simulink model "buck_N"  (R2023a)
settings: Solver=ode4  StartTime=0.0  StopTime=Tsin  FixedStep=Ts  RelTol=1e-3
values from neighbouring files (symbols this model uses):
  C1 = 100e-6*(1.0)    (= 0.0001)    [ripp_buck2.m]
  kd = x3    [ripp_buck2.m]
  ki = x2    [ripp_buck2.m]
  kp = x1    [ripp_buck2.m]
  L1 = 1e-3*(1.0)    (= 0.001)    [ripp_buck2.m]
  R1 = 6    [ripp_buck2.m]
  Ref = 3    [ripp_buck2.m]
  Ts = H.SettlingTime    [HHbuck.m]    (also in ripp_buck2.m)
  Tsin = 0.01    [ripp_buck2.m]
  Vg = 36    [ripp_buck2.m]
libraries: simulink x3, spsSeriesRLCBranchLib x3, spsControlledCurrentSourceLib x1, spsCurrentMeasurementLib x1, spsDCVoltageSourceLib x1, spsDiodeLib x1, spsMosfetLib x1, spsPWMGeneratorDCDCLib x1, spsVoltageMeasurementLib x1, spspowerguiLib x1
settings Model: SimulationMode=accelerator  Creator=danie  LastModifiedBy=Daniel
settings DataIOCC: ReturnWorkspaceOutputs=off
settings ModelReferenceCC: EnableRefExpFcnMdlSchedulingChecks=on

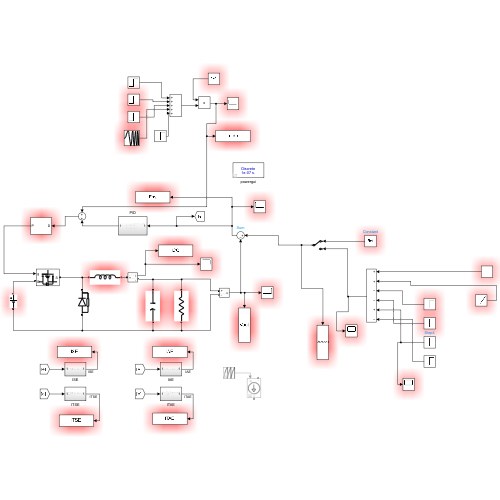
[thumbnail: Simulink's stored preview of the top-level diagram]
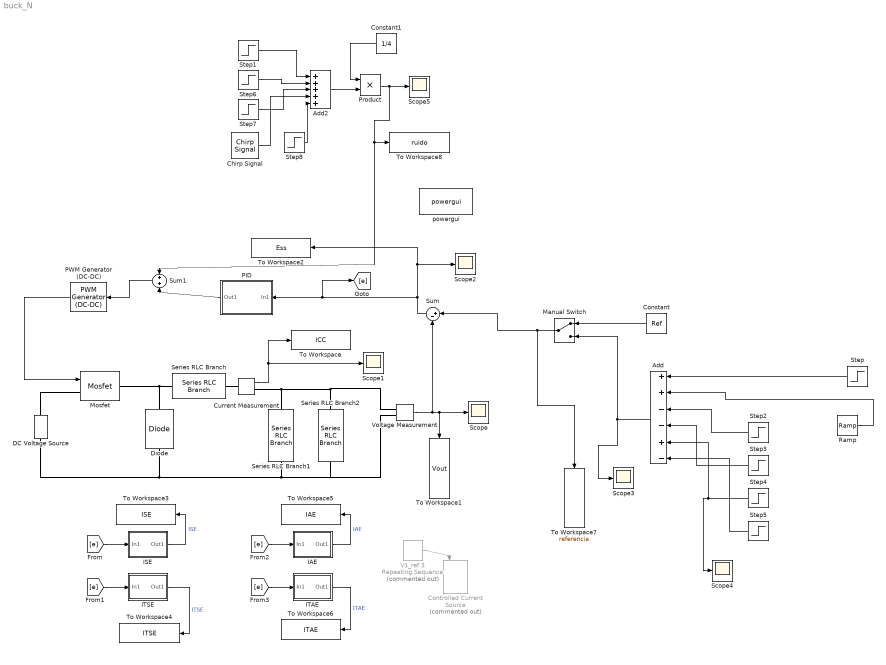
== system buck_N ==
  Add : Sum  Inputs=++--+-
  Add2 : Sum  Inputs=+++++
  Chirp Signal : simulink/Sources/Chirp Signal  f1=1e2  T=Tsin  f2=5e3
  Constant : Constant  Value=Ref  SampleTime=Ts
  Constant1 : Constant  Value=1/4  SampleTime=Ts
  Controlled Current Source : spsControlledCurrentSourceLib/Controlled Current Source  Commented=on  Initialize=off  Source_Type=AC  Amplitude=0  Phase=0  Frequency=0  Measurements=None
  Current Measurement : spsCurrentMeasurementLib/Current Measurement  PhasorSimulation=off  OutputType=Complex  PSBequivalent=0
  DC Voltage Source : spsDCVoltageSourceLib/DC Voltage Source  Amplitude=Vg  Measurements=None
  Diode : spsDiodeLib/Diode  Ron=0.001  Lon=0  Vf=0.8  IC=0  UseSnubber=0  Rs=500  Cs=250e-9  Measurements=off
  IAE : Subsystem
  ISE : Subsystem
  ITAE : Subsystem
  ITSE : Subsystem
  Manual Switch : ManualSwitch
  Mosfet : spsMosfetLib/Mosfet  Ron=0.1  Lon=0  Rd=0.01  Vfd=0  IC=0  Rs=1e5  Cs=inf  Measurements=off
  PID : Subsystem
  PWM Generator (DC-DC) : spsPWMGeneratorDCDCLib/PWM Generator (DC-DC)  Fsw=F  Ts=Ts
  Product : Product
  Ramp : simulink/Sources/Ramp  slope=100  start=Tsin/2  InitialOutput=0
  Scope{,1..5} (6 alike) : Scope
  Series RLC Branch : spsSeriesRLCBranchLib/Series RLC Branch  LConnTagsString=__new0  RConnTagsString=__new0  BranchType=L  Resistance=1  Inductance=L1  SetiL0=off  InitialCurrent=0  Capacitance=1e-6  Setx0=off  InitialVoltage=0  Measurements=None
  Series RLC Branch1 : spsSeriesRLCBranchLib/Series RLC Branch  LConnTagsString=__new0  RConnTagsString=__new0  BranchType=C  Resistance=1  Inductance=1e-3  SetiL0=off  InitialCurrent=0  Capacitance=C1  Setx0=off  InitialVoltage=0  Measurements=None
  Series RLC Branch2 : spsSeriesRLCBranchLib/Series RLC Branch  LConnTagsString=__new0  RConnTagsString=__new0  BranchType=R  Resistance=R1  Inductance=1e-3  SetiL0=off  InitialCurrent=0  Capacitance=1e-6  Setx0=off  InitialVoltage=0  Measurements=None
  Step : Step  Time=Tsin/5  After=3  SampleTime=0
  Step1 : Step  Time=0  After=0.5  SampleTime=0
  Step2 : Step  Time=Tsin/3  After=2  SampleTime=0
  Step3 : Step  Time=Tsin/2  After=-3  SampleTime=0
  Step4 : Step  Time=0  After=3  SampleTime=0
  Step5 : Step  Time=0.04  After=3  SampleTime=0
  Step6 : Step  Time=Tsin/4  After=0.3  SampleTime=0
  Step7 : Step  Time=Tsin/2  After=0.4  SampleTime=0
  Step8 : Step  Time=0  SampleTime=0
  Sum : Sum  Inputs=|+-
  Sum1 : Sum
  To Workspace : ToWorkspace  VariableName=ICC  SaveFormat=Structure With Time  SampleTime=Ts
  To Workspace1 : ToWorkspace  VariableName=Vout  SaveFormat=Structure With Time  SampleTime=Ts
  To Workspace2 : ToWorkspace  VariableName=Ess  SaveFormat=Structure With Time  SampleTime=Ts
  To Workspace3 : ToWorkspace  VariableName=ISE  SaveFormat=Structure With Time  SampleTime=Ts
  To Workspace4 : ToWorkspace  VariableName=ITSE  SaveFormat=Structure With Time  SampleTime=Ts
  To Workspace5 : ToWorkspace  VariableName=IAE  SaveFormat=Structure With Time  SampleTime=Ts
  To Workspace6 : ToWorkspace  VariableName=ITAE  SaveFormat=Structure With Time  SampleTime=Ts
  To Workspace7 : ToWorkspace  VariableName=referencia  SaveFormat=Structure With Time  SampleTime=Ts
  To Workspace8 : ToWorkspace  VariableName=ruido  SaveFormat=Structure With Time  SampleTime=Ts
  V1_ref 3 : simulink/Sources/Repeating Sequence  Commented=on  rep_seq_t=[0 0.015/5 0.015/3 0.015/2 ]  rep_seq_y="[0 6 8 10  ]"
  Voltage Measurement : spsVoltageMeasurementLib/Voltage Measurement  PhasorSimulation=off  OutputType=Complex  PSBequivalent=0
  powergui : spspowerguiLib/powergui  Priority=1  SimulationMode=Discrete  SampleTime=Ts  frequency=60  Iterations=50  frequencyindice=0  Pbase=100e6  ErrMax=1e-4  UnitsV=kV  UnitsW=MW  buscounter=0  FunctionMessages=off  echomessages=off  EnableUseOfTLC=off  CurrentSourceSwitches=off  DisableSnubberDevices=off  DisableRonSwitches=off  DisableVfSwitches=off  DisplayEquations=off  AutomaticDiscreteSolvers=off  SolverType=Tustin/Backward Euler (TBE)  Interpol=off  ExternalGateDelay=off  methode=off  Ts=100  x0status=blocks  SPID=on  SwTol=0  HookPort=off  NonlinearTolerance=1e-4  nMaxIteration=100  ContinueOnMaxIteration=off  RestoreLinks=warning  ResistiveCurrentMeasurement=off  Frange=[0:2:500]  Ylog=off  Xlog=on  ShowGrid=off  save=off  variable=ZData  structure=0  ZoomFFT=off  StartTime=0.0  cycles=1  DisplayStyle=1  fundamental=60  FreqAxis=off  MaxFrequency=1000  frequencyindicesteady=1  RmsSteady=1  display=off
  wires:
  Voltage Measurement/1 -> Scope/1, To Workspace1/1, Sum/2
  Current Measurement/1 -> To Workspace/1, Scope1/1
  PWM Generator (DC-DC)/1 -> Mosfet/1
  V1_ref 3/1 -> Controlled Current Source/1
  Sum/1 -> To Workspace2/1, Scope2/1, [e], PID/1(In1)
  [e] -> ITSE/1(In1)
  ISE/1(Out1) -> To Workspace3/1  "ISE"
  IAE/1(Out1) -> To Workspace5/1  "IAE"
  ITSE/1(Out1) -> To Workspace4/1  "ITSE"
  ITAE/1(Out1) -> To Workspace6/1  "ITAE"
  [e] -> ISE/1(In1)
  [e] -> ITAE/1(In1)
  [e] -> IAE/1(In1)
  Manual Switch/1 -> To Workspace7/1, Sum/1
  Constant/1 -> Manual Switch/1
  Add/1 -> Scope3/1, Manual Switch/2
  Step/1 -> Add/1
  Ramp/1 -> Add/2
  Step2/1 -> Add/3
  Step3/1 -> Add/4
  Step4/1 -> Add/5, Scope4/1
  Step5/1 -> Add/6
  Step1/1 -> Add2/1
  Step6/1 -> Add2/2
  Step7/1 -> Add2/3
  Chirp Signal/1 -> Add2/4
  PID/1(Out1) -> Sum1/2
  Sum1/1 -> PWM Generator (DC-DC)/1
  Step8/1 -> Add2/5
  Add2/1 -> Product/2
  Product/1 -> Sum1/1, To Workspace8/1, Scope5/1
  Constant1/1 -> Product/1
  connections:
  Mosfet/LConn1 -- DC Voltage Source/RConn1
  Mosfet/RConn1 -- Series RLC Branch/RConn1 -- Diode/RConn1
  DC Voltage Source/LConn1 -- Voltage Measurement/LConn2 -- Series RLC Branch2/RConn1 -- Series RLC Branch1/RConn1 -- Diode/LConn1
  Series RLC Branch/LConn1 -- Current Measurement/LConn1
  Voltage Measurement/LConn1 -- Series RLC Branch2/LConn1 -- Current Measurement/RConn1 -- Series RLC Branch1/LConn1

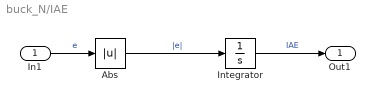
== system buck_N/IAE ==
  In1 : Inport
  Abs : Abs  SaturateOnIntegerOverflow=off
  Integrator : Integrator
  Out1 : Outport
  wires:
  Integrator/1 -> Out1/1  "IAE"
  In1/1 -> Abs/1  "e"
  Abs/1 -> Integrator/1  "|e|"

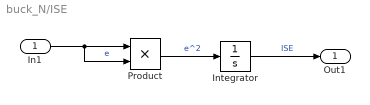
== system buck_N/ISE ==
  In1 : Inport
  Integrator : Integrator
  Product : Product
  Out1 : Outport
  wires:
  In1/1 -> Product/2, Product/1  "e"
  Product/1 -> Integrator/1  "e^2"
  Integrator/1 -> Out1/1  "ISE"

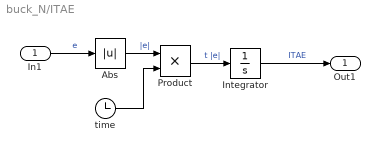
== system buck_N/ITAE ==
  In1 : Inport
  Abs : Abs  SaturateOnIntegerOverflow=off
  Integrator : Integrator
  Product : Product
  time : Clock
  Out1 : Outport
  wires:
  In1/1 -> Abs/1  "e"
  Integrator/1 -> Out1/1  "ITAE"
  time/1 -> Product/2
  Abs/1 -> Product/1  "|e|"
  Product/1 -> Integrator/1  "t |e|"

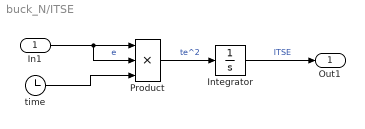
== system buck_N/ITSE ==
  In1 : Inport
  Integrator : Integrator
  Product : Product  Inputs=3
  time : Clock
  Out1 : Outport
  wires:
  Integrator/1 -> Out1/1  "ITSE"
  In1/1 -> Product/1, Product/2  "e"
  time/1 -> Product/3
  Product/1 -> Integrator/1  "te^2"

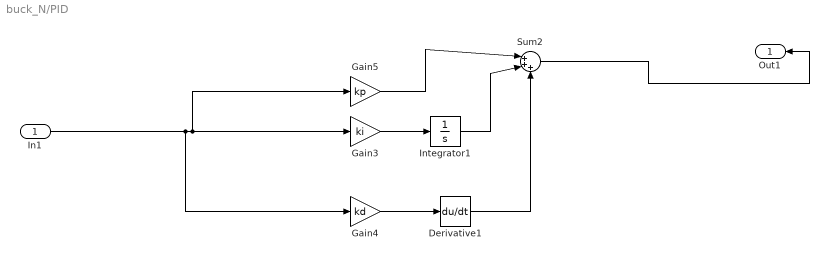
== system buck_N/PID ==
  In1 : Inport
  Derivative1 : Derivative  CoefficientInTFapproximation=10
  Gain3 : Gain  Gain=ki
  Gain4 : Gain  Gain=kd
  Gain5 : Gain  Gain=kp
  Integrator1 : Integrator
  Sum2 : Sum  Inputs=|+++
  Out1 : Outport
  wires:
  Gain5/1 -> Sum2/1
  In1/1 -> Gain4/1, Gain3/1, Gain5/1
  Gain3/1 -> Integrator1/1
  Sum2/1 -> Out1/1
  Derivative1/1 -> Sum2/3
  Integrator1/1 -> Sum2/2
  Gain4/1 -> Derivative1/1
